simulink model "induction_test"  (R2023b)
settings: Solver=VariableStepAuto  StartTime=0.0  StopTime=25  FixedStep=0.001  RelTol=1e-5
undefined symbols (not defined in the file): amplitude
libraries: autolibim x1
settings Model: Creator=root  LastModifiedBy=root

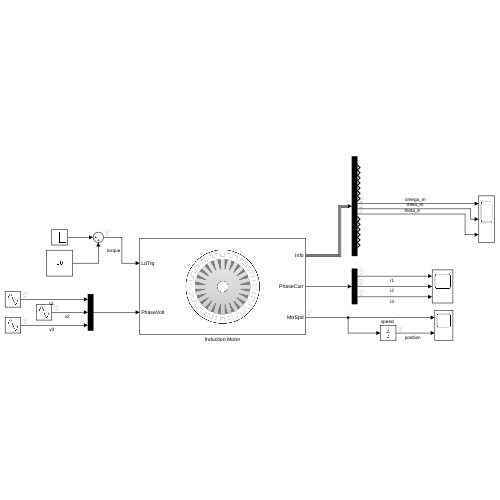
[thumbnail: Simulink's stored preview of the top-level diagram]
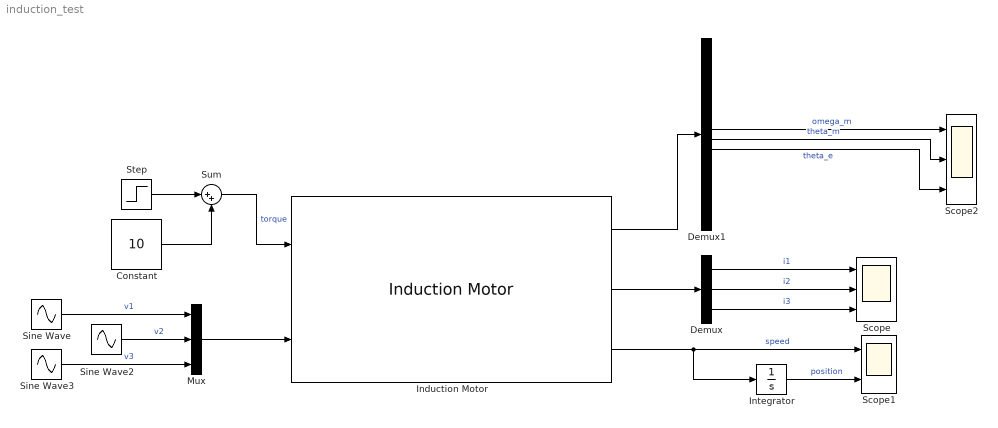
== system induction_test ==
  Constant : Constant  Value=10
  Demux : Demux  Outputs=3
  Demux1 : Demux  Outputs=16
  Induction Motor : autolibim/Induction Motor  sim_type=Continuous  Ts=0.001  port_config=Torque  P=2  Zs=[1.77 0.0139]  Zr="[1.34  0.0121]"  Lm=0.3687  mechanical=[0.001 0 0]  theta_init=0  omega_init=0  RefBlkName='autolibim/Induction Motor'  aMode=1
      settings: LibrarySourceBlock=autolibemachines/Induction Motor
  Integrator : Integrator
  Mux : Mux  Inputs=3
  Scope : Scope  NumInputPorts=3
  Scope1 : Scope  NumInputPorts=2
  Scope2 : Scope  NumInputPorts=3
  Sine Wave : Sin  Amplitude=amplitude  Frequency=50*(pi/180)  SampleTime=0
  Sine Wave2 : Sin  Amplitude=amplitude  Frequency=50*(pi/180)  Phase=(2*pi)/3  SampleTime=0
  Sine Wave3 : Sin  Amplitude=amplitude  Frequency=50*(pi/180)  Phase=(4*pi)/3  SampleTime=0
  Step : Step  Time=10  After=-250  SampleTime=0
  Sum : Sum  Inputs=|++
  wires:
  Mux/1 -> Induction Motor/2
  Sine Wave/1 -> Mux/1  "v1"
  Sine Wave2/1 -> Mux/2  "v2"
  Sine Wave3/1 -> Mux/3  "v3"
  Induction Motor/2 -> Demux/1
  Demux/1 -> Scope/1  "i1"
  Demux/2 -> Scope/2  "i2"
  Demux/3 -> Scope/3  "i3"
  Constant/1 -> Sum/2
  Step/1 -> Sum/1
  Sum/1 -> Induction Motor/1  "torque"
  Induction Motor/3 -> Integrator/1, Scope1/1  "speed"
  Integrator/1 -> Scope1/2  "position"
  Induction Motor/1 -> Demux1/1
  Demux1/9 -> Scope2/2  "theta_m"
  Demux1/10 -> Scope2/3  "theta_e"
  Demux1/8 -> Scope2/1  "omega_m"
